simulink model "car_simulator_velocity"  (R2021a)
settings: Solver=ode45  StartTime=0.0  StopTime=25  RelTol=1e-4
model workspace (MAT data in the model file):
  Freq = 1
values from neighbouring files (symbols this model uses):
  actuator_param = [mu_steer wn_steer csi_steer tau_steer mu_speed wn_speed csi_speed tau_speed]    [test_singletrack_fialaws_ideal.m]    (also in test_singletrack_force_fialawos_ideal.m = [mu_steer wn_steer csi_steer tau_steer mu_force wn_force csi; test_singletrack_force_fialawos_real.m = [mu_steer wn_steer csi_steer tau_steer mu_force wn_force csi; test_singletrack_force_fialaws_ideal.m = [mu_steer wn_steer csi_steer tau_steer mu_force wn_force csi; test_singletrack_force_fialaws_real.m = [mu_steer wn_steer csi_steer tau_steer mu_force wn_force csi)
  car_param = [a b m mu Cf Cr Iz]    [test_singletrack_fialaws_ideal.m]    (also in test_singletrack_force_fialawos_ideal.m; test_singletrack_force_fialawos_real.m; test_singletrack_force_fialaws_ideal.m; test_singletrack_force_fialaws_real.m)
  initial_state = [vy0 r0 psi0 x0 y0]    [test_singletrack_fialaws_ideal.m]    (also in test_singletrack_force_fialawos_ideal.m = [vx0 vy0 r0 psi0 x0 y0]; test_singletrack_force_fialawos_real.m = [vx0 vy0 r0 psi0 x0 y0]; test_singletrack_force_fialaws_ideal.m = [vx0 vy0 r0 psi0 x0 y0]; test_singletrack_force_fialaws_real.m = [vx0 vy0 r0 psi0 x0 y0])
  speed_ref = timeseries(ode_res.speed_ref,ode_res.t)    [test_singletrack_fialaws_ideal.m]    (also in test_singletrack_linear_real.m; test_singletrack_velocity_fialawos_ideal.m; test_singletrack_velocity_fialawos_real.m; test_singletrack_velocity_fialaws_ideal.m)
  steer_ref = timeseries(ode_res.steer_ref,ode_res.t)    [test_singletrack_fialaws_ideal.m]    (also in test_singletrack_force_fialawos_ideal.m; test_singletrack_force_fialawos_real.m; test_singletrack_force_fialaws_ideal.m; test_singletrack_force_fialaws_real.m)
  Ts = ode_res.t(2)-ode_res.t(1)    [test_singletrack_fialaws_ideal.m]    (also in test_singletrack_force_fialawos_ideal.m; test_singletrack_force_fialawos_real.m; test_singletrack_force_fialaws_ideal.m; test_singletrack_force_fialaws_real.m)
  tyre_model = 1    [test_singletrack_fialaws_ideal.m]    (also in test_singletrack_force_fialawos_ideal.m = 2; test_singletrack_force_fialawos_real.m = 2; test_singletrack_force_fialaws_ideal.m; test_singletrack_force_fialaws_real.m)
settings Model: Creator=bascetta  LastModifiedBy=bascetta
settings SolverCC: AlgebraicLoopSolver=TrustRegion  DecoupledContinuousIntegration=on
settings DataIOCC: SaveOutput=off  SignalLogging=off  DSMLogging=off  SaveTime=off  ReturnWorkspaceOutputs=off
settings DebuggingCC: ReadBeforeWriteMsg=DisableAll  WriteAfterWriteMsg=DisableAll  WriteAfterReadMsg=DisableAll  MultiTaskDSMMsg=none  SFMachineParentedDataDiag=warning  ArithmeticOperatorsInVariantConditions=warning
settings ModelReferenceCC: UpdateModelReferenceTargets=IfOutOfDate
settings SFSimCC: SFSimEcho=off  SimUseLocalCustomCode=off  CustomCodeUndefinedFunction=UseInterfaceOnly
settings RTWCC: RTWUseLocalCustomCode=off

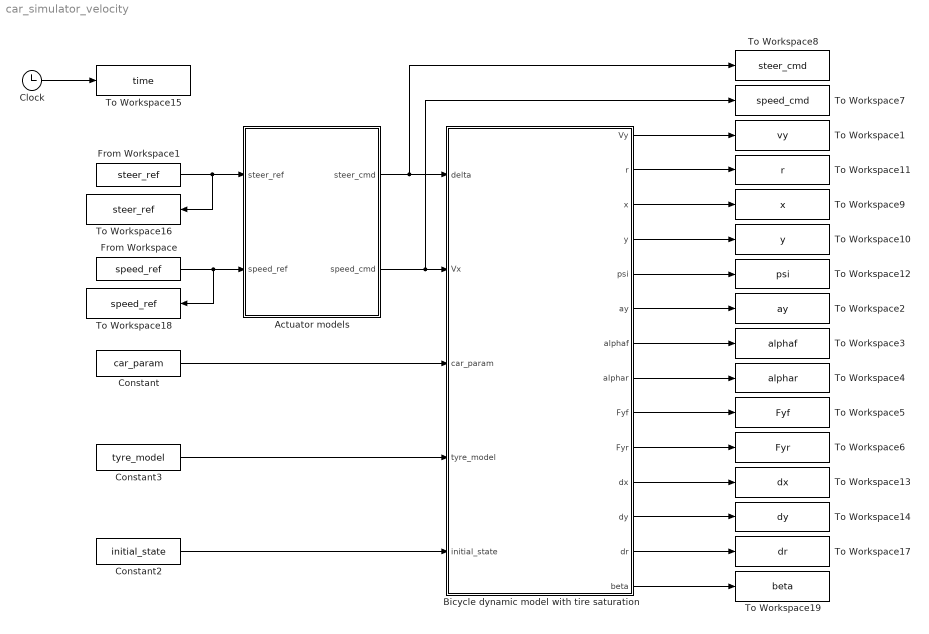
== system car_simulator_velocity ==
  Actuator models : Subsystem  mask{mu_steer=actuator_param(1), wn_steer=actuator_param(2), csi_steer=actuator_param(3), tau_steer=actuator_param(4), steer_initial=steer_ref.Data(1), mu_speed=actuator_param(5), wn_speed=actuator_param(6), csi_speed=actuator_param(7), tau_speed=actuator_param(8), speed_initial=speed_ref.Data(1)}
      mask prompts: mu_steer "Gain"; wn_steer "Natural frequency"; csi_steer "Damping"; tau_steer "Delay"; steer_initial "Initial value"; mu_speed "Gain"; wn_speed "Natural frequency"; csi_speed "Damping"; tau_speed "Delay"; speed_initial "Initial value"
      mask DialogControl Container3 Prompt: Steer actuator parameters
      mask DialogControl Container4 Prompt: Speed actuator parameters
  Bicycle dynamic model with tire saturation : Subsystem
  Clock : Clock
  Constant : Constant  Value=car_param
  Constant2 : Constant  Value=initial_state
  Constant3 : Constant  Value=tyre_model
  From Workspace : FromWorkspace  VariableName=speed_ref
  From Workspace1 : FromWorkspace  VariableName=steer_ref
  To Workspace1 : ToWorkspace  VariableName=vy  SampleTime=Ts
      settings: Save2DSignal=2-D array (concatenate along first dimension)
  To Workspace10 : ToWorkspace  VariableName=y  SampleTime=Ts
      settings: Save2DSignal=2-D array (concatenate along first dimension)
  To Workspace11 : ToWorkspace  VariableName=r  SampleTime=Ts
      settings: Save2DSignal=2-D array (concatenate along first dimension)
  To Workspace12 : ToWorkspace  VariableName=psi  SampleTime=Ts
      settings: Save2DSignal=2-D array (concatenate along first dimension)
  To Workspace13 : ToWorkspace  VariableName=dx  SampleTime=Ts
      settings: Save2DSignal=2-D array (concatenate along first dimension)
  To Workspace14 : ToWorkspace  VariableName=dy  SampleTime=Ts
      settings: Save2DSignal=2-D array (concatenate along first dimension)
  To Workspace15 : ToWorkspace  VariableName=time  SampleTime=Ts
      settings: Save2DSignal=2-D array (concatenate along first dimension)
  To Workspace16 : ToWorkspace  VariableName=steer_ref  SampleTime=Ts
      settings: Save2DSignal=2-D array (concatenate along first dimension)
  To Workspace17 : ToWorkspace  VariableName=dr  SampleTime=Ts
      settings: Save2DSignal=2-D array (concatenate along first dimension)
  To Workspace18 : ToWorkspace  VariableName=speed_ref  SampleTime=Ts
      settings: Save2DSignal=2-D array (concatenate along first dimension)
  To Workspace19 : ToWorkspace  VariableName=beta  SampleTime=Ts
      settings: Save2DSignal=2-D array (concatenate along first dimension)
  To Workspace2 : ToWorkspace  VariableName=ay  SampleTime=Ts
      settings: Save2DSignal=2-D array (concatenate along first dimension)
  To Workspace3 : ToWorkspace  VariableName=alphaf  SampleTime=Ts
      settings: Save2DSignal=2-D array (concatenate along first dimension)
  To Workspace4 : ToWorkspace  VariableName=alphar  SampleTime=Ts
      settings: Save2DSignal=2-D array (concatenate along first dimension)
  To Workspace5 : ToWorkspace  VariableName=Fyf  SampleTime=Ts
      settings: Save2DSignal=2-D array (concatenate along first dimension)
  To Workspace6 : ToWorkspace  VariableName=Fyr  SampleTime=Ts
      settings: Save2DSignal=2-D array (concatenate along first dimension)
  To Workspace7 : ToWorkspace  VariableName=speed_cmd  SampleTime=Ts
      settings: Save2DSignal=2-D array (concatenate along first dimension)
  To Workspace8 : ToWorkspace  VariableName=steer_cmd  SampleTime=Ts
      settings: Save2DSignal=2-D array (concatenate along first dimension)
  To Workspace9 : ToWorkspace  VariableName=x  SampleTime=Ts
      settings: Save2DSignal=2-D array (concatenate along first dimension)
  wires:
  Bicycle dynamic model with tire saturation/1(Vy) -> To Workspace1/1
  Bicycle dynamic model with tire saturation/2(r) -> To Workspace11/1
  Bicycle dynamic model with tire saturation/6(ay) -> To Workspace2/1
  Bicycle dynamic model with tire saturation/7(alphaf) -> To Workspace3/1
  Bicycle dynamic model with tire saturation/8(alphar) -> To Workspace4/1
  Bicycle dynamic model with tire saturation/9(Fyf) -> To Workspace5/1
  Bicycle dynamic model with tire saturation/10(Fyr) -> To Workspace6/1
  Constant/1 -> Bicycle dynamic model with tire saturation/3(car_param)
  Constant2/1 -> Bicycle dynamic model with tire saturation/5("initial_state ")
  Constant3/1 -> Bicycle dynamic model with tire saturation/4(tyre_model)
  Actuator models/1(steer_cmd) -> To Workspace8/1, Bicycle dynamic model with tire saturation/1(delta)
  Actuator models/2(speed_cmd) -> To Workspace7/1, Bicycle dynamic model with tire saturation/2(Vx)
  From Workspace/1 -> To Workspace18/1, Actuator models/2(speed_ref)
  From Workspace1/1 -> To Workspace16/1, Actuator models/1(steer_ref)
  Bicycle dynamic model with tire saturation/3(x) -> To Workspace9/1
  Bicycle dynamic model with tire saturation/4(y) -> To Workspace10/1
  Bicycle dynamic model with tire saturation/5(psi) -> To Workspace12/1
  Bicycle dynamic model with tire saturation/11(dx) -> To Workspace13/1
  Bicycle dynamic model with tire saturation/12(dy) -> To Workspace14/1
  Clock/1 -> To Workspace15/1
  Bicycle dynamic model with tire saturation/13(dr) -> To Workspace17/1
  Bicycle dynamic model with tire saturation/14(beta) -> To Workspace19/1

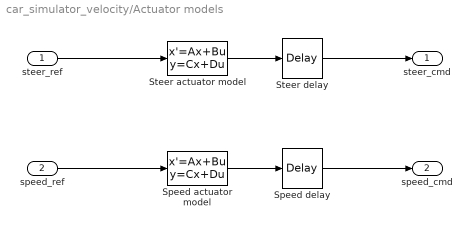
== system car_simulator_velocity/Actuator models ==
  steer_ref : Inport
  speed_ref : Inport  Port=2
  Speed actuator model : StateSpace  A=[0, 1; -wn_speed^2, -2*csi_speed*wn_speed]  B=[0; mu_speed*wn_speed^2]  C=[1, 0]  D=0  InitialCondition=[speed_initial, 0]
  Speed delay : TransportDelay  DelayTime=tau_speed  InitialOutput=speed_initial
  Steer actuator model : StateSpace  A=[0, 1; -wn_steer^2, -2*csi_steer*wn_steer]  B=[0; mu_steer*wn_steer^2]  C=[1, 0]  D=0  InitialCondition=[steer_initial, 0]
  Steer delay : TransportDelay  DelayTime=tau_steer  InitialOutput=steer_initial
  steer_cmd : Outport
  speed_cmd : Outport  Port=2
  wires:
  speed_ref/1 -> Speed actuator model/1
  Steer actuator model/1 -> Steer delay/1
  Speed actuator model/1 -> Speed delay/1
  steer_ref/1 -> Steer actuator model/1
  Steer delay/1 -> steer_cmd/1
  Speed delay/1 -> speed_cmd/1

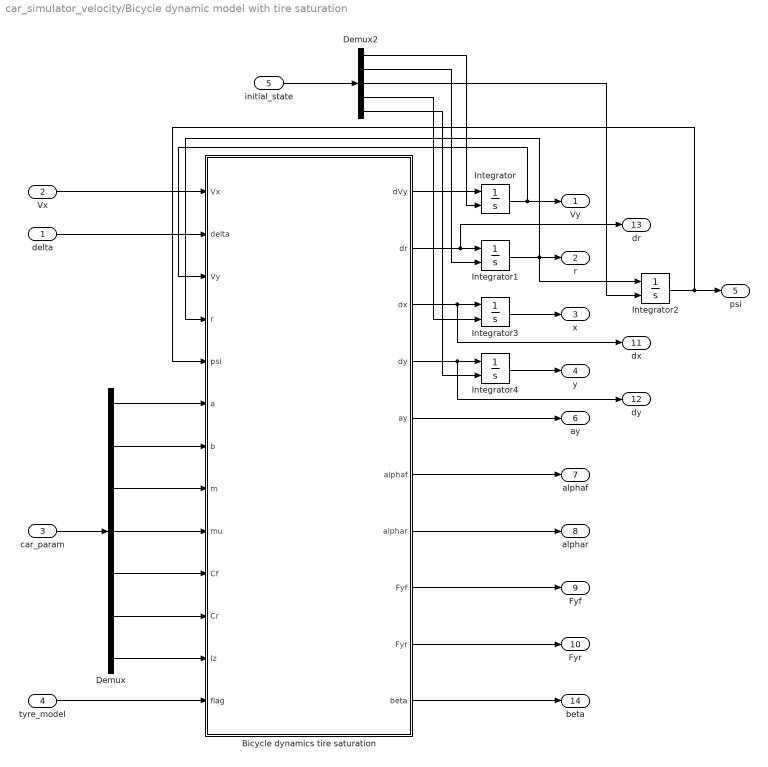
== system car_simulator_velocity/Bicycle dynamic model with tire saturation ==
  delta : Inport
  Vx : Inport  Port=2
  car_param : Inport  Port=3
  tyre_model : Inport  Port=4
  "initial_state " : Inport  Port=5
  Bicycle dynamics tire saturation : MATLAB Function  TreatAsAtomicUnit=on
  Demux : Demux  Outputs=7
  Demux2 : Demux  Outputs=5
  Integrator{,1..4} (5 alike) : Integrator  InitialConditionSource=external
  Vy : Outport
  r : Outport  Port=2
  x : Outport  Port=3
  y : Outport  Port=4
  psi : Outport  Port=5
  ay : Outport  Port=6
  alphaf : Outport  Port=7
  alphar : Outport  Port=8
  Fyf : Outport  Port=9
  Fyr : Outport  Port=10
  dx : Outport  Port=11
  dy : Outport  Port=12
  dr : Outport  Port=13
  beta : Outport  Port=14
  wires:
  Vx/1 -> Bicycle dynamics tire saturation/1(Vx)
  delta/1 -> Bicycle dynamics tire saturation/2(delta)
  Bicycle dynamics tire saturation/1(dVy) -> Integrator/1
  Bicycle dynamics tire saturation/2(dr) -> dr/1, Integrator1/1
  Integrator/1 -> Vy/1, Bicycle dynamics tire saturation/3(Vy)
  Integrator1/1 -> Bicycle dynamics tire saturation/4(r), r/1, Integrator2/1
  Bicycle dynamics tire saturation/5(ay) -> ay/1
  Bicycle dynamics tire saturation/6(alphaf) -> alphaf/1
  Bicycle dynamics tire saturation/7(alphar) -> alphar/1
  Bicycle dynamics tire saturation/8(Fyf) -> Fyf/1
  Bicycle dynamics tire saturation/9(Fyr) -> Fyr/1
  car_param/1 -> Demux/1
  Demux/1 -> Bicycle dynamics tire saturation/6(a)
  Demux/2 -> Bicycle dynamics tire saturation/7(b)
  Demux/3 -> Bicycle dynamics tire saturation/8(m)
  Demux/4 -> Bicycle dynamics tire saturation/9(mu)
  "initial_state "/1 -> Demux2/1
  Demux2/1 -> Integrator/2
  Demux2/2 -> Integrator1/2
  tyre_model/1 -> Bicycle dynamics tire saturation/13(flag)
  Demux/5 -> Bicycle dynamics tire saturation/10(Cf)
  Demux/6 -> Bicycle dynamics tire saturation/11(Cr)
  Demux/7 -> Bicycle dynamics tire saturation/12(Iz)
  Bicycle dynamics tire saturation/3(dx) -> dx/1, Integrator3/1
  Bicycle dynamics tire saturation/4(dy) -> dy/1, Integrator4/1
  Integrator3/1 -> x/1
  Integrator4/1 -> y/1
  Demux2/3 -> Integrator2/2
  Demux2/4 -> Integrator3/2
  Demux2/5 -> Integrator4/2
  Integrator2/1 -> Bicycle dynamics tire saturation/5(psi), psi/1
  Bicycle dynamics tire saturation/10(beta) -> beta/1

== matlab function car_simulator_velocity/Bicycle dynamic model with tire saturation/Bicycle dynamics tire saturation ==
  data: dVy output; Vx input; dr output; dx output; dy output; delta input; Vy input; r input; psi input; a input; b input; m input; mu input; Cf input; Cr input; Iz input; ay output; alphaf output; alphar output; Fyf output; Fyr output; flag input; beta output
function [dVy,dr,dx,dy,ay,alphaf,alphar,Fyf,Fyr,beta]  = bicycle_dynamics(Vx, delta, Vy, r, psi, a, b, m, mu, Cf, Cr, Iz, flag)

Fzf = m*9.81*b/(a+b);
Fzr = m*9.81*a/(a+b);

if (abs(Vx)<=0.01)
    alphaf = 0;
    alphar = 0;
else
    alphaf = atan((Vy+a*r)/Vx)-delta;
    alphar = atan((Vy-b*r)/Vx);
end

zf = tan(alphaf);
zr = tan(alphar);

zf_sl = 3*mu*Fzf/Cf;
zr_sl = 3*mu*Fzr/Cr;

switch flag
    case 0 % Linear tyre model
        Fyf = -Cf*alphaf;
        Fyr = -Cr*alphar;
    case 1 % Fiala model with saturation
        if (abs(zf)<zf_sl)
            Fyf = Cf*zf*(-1+abs(zf)/zf_sl-zf^2/(3*zf_sl^2));
        else
            Fyf = -mu*Fzf*sign(alphaf);
        end
        if (abs(zr)<zr_sl)
            Fyr = Cr*zr*(-1+abs(zr)/zr_sl-zr^2/(3*zr_sl^2));
        else
            Fyr = -mu*Fzr*sign(alphar);
        end
    case 2 % Fiala model without saturation
        Fyf = Cf*zf*(-1+abs(zf)/zf_sl-zf^2/(3*zf_sl^2));
        Fyr = Cr*zr*(-1+abs(zr)/zr_sl-zr^2/(3*zr_sl^2));
    otherwise
        Fyf = 0;
        Fyr = 0;
end

dr  = (a*Fyf*cos(delta)-b*Fyr)/Iz;
dVy = (Fyf*cos(delta)+Fyr)/m-r*Vx;
ay  = dVy+r*Vx;

R_psi = [cos(psi), -sin(psi); sin(psi), cos(psi)];
dx  = R_psi(1,1:2)*[Vx; Vy];
dy  = R_psi(2,1:2)*[Vx; Vy];

if (abs(Vx)<=0.01)
    beta = 0;
else
    beta = atan2(Vy,Vx);
end
